simulink model "zd_model"  (Simulink 4.00)
settings: Solver=ode45  SolverMode=SingleTasking  StartTime=0.0  StopTime=T  FixedStep=.001  RelTol=1e-5  AbsTol=1e-6
values from neighbouring files (symbols this model uses):
  z0 = zd_project(x0)    [main_zd.m]    (also in sim_zd_cc.m = zd_project_cc(x0(1:10)'))
undefined symbols (not defined in the file or in its folder): x_0
settings Model: Creator=ewesterv  LastModifiedBy=ewesterv  TimeSaveName=t  LimitDataPoints=off  BlockReductionOpt=off

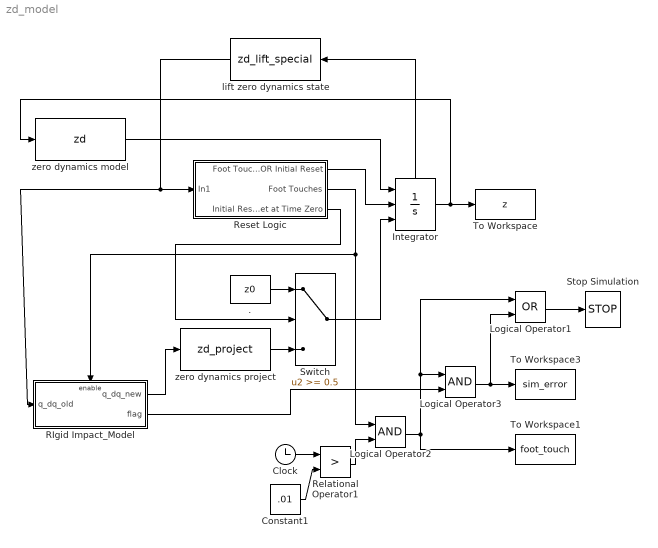
== system zd_model ==
  . : Constant  Value=z0
  Clock : Clock
      settings: DisplayTime=off  Decimation=10
  Constant1 : Constant  Value=.01
  Integrator : Integrator  ExternalReset=rising  InitialConditionSource=external  InitialCondition=x_0  LimitOutput=off  UpperSaturationLimit=inf  LowerSaturationLimit=-inf  ShowSaturationPort=off  ShowStatePort=on  AbsoluteTolerance=auto
  Logical Operator1 : Logic  Operator=OR  Inputs=2
  Logical Operator2 : Logic  Operator=AND  Inputs=2
  Logical Operator3 : Logic  Operator=AND  Inputs=2
  RIgid Impact_Model : Subsystem  TreatAsAtomicUnit=on
      settings: RTWFcnNameOpts=Auto  RTWFileNameOpts=Auto
  Relational Operator1 : RelationalOperator  Operator=>
  Reset Logic : Subsystem
      settings: RTWFcnNameOpts=Auto  RTWFileNameOpts=Auto
  Stop Simulation : Stop
  Switch : Switch  Threshold=0.5
  To Workspace : ToWorkspace  VariableName=z  SampleTime=-1  SaveFormat=Array
  To Workspace1 : ToWorkspace  VariableName=foot_touch  SampleTime=-1  SaveFormat=Array
  To Workspace3 : ToWorkspace  VariableName=sim_error  SampleTime=-1  SaveFormat=Array
  lift zero dynamics state : MATLABFcn  Orientation=left  MATLABFcn=zd_lift_special  OutputDimensions=10  OutputSignalType=auto  Output1D=off
  zero dynamics model : MATLABFcn  MATLABFcn=zd  OutputDimensions=2  OutputSignalType=auto  Output1D=on
  zero dynamics project : MATLABFcn  MATLABFcn=zd_project  OutputDimensions=2  OutputSignalType=auto  Output1D=on
  wires:
  Relational Operator1/1 -> Logical Operator2/2
  RIgid Impact_Model/2(flag) -> Logical Operator3/2
  Clock/1 -> Relational Operator1/1
  Integrator/1 -> To Workspace/1, zero dynamics model/1
  Reset Logic/2(Foot Touches) -> Logical Operator2/1, RIgid Impact_Model/Enable
  ./1 -> Switch/1
  Reset Logic/3(Initial Reset at Time Zero) -> Switch/2
  Switch/1 -> Integrator/3
  Reset Logic/1(Foot Touch OR Initial Reset) -> Integrator/2
  zero dynamics model/1 -> Integrator/1
  Constant1/1 -> Relational Operator1/2
  Logical Operator3/1 -> To Workspace3/1, Logical Operator1/2
  Integrator/State -> lift zero dynamics state/1
  lift zero dynamics state/1 -> Reset Logic/1(In1), RIgid Impact_Model/1(q_dq_old)
  RIgid Impact_Model/1(q_dq_new) -> zero dynamics project/1
  zero dynamics project/1 -> Switch/3
  Logical Operator1/1 -> Stop Simulation/1
  Logical Operator2/1 -> Logical Operator1/1, Logical Operator3/1, To Workspace1/1

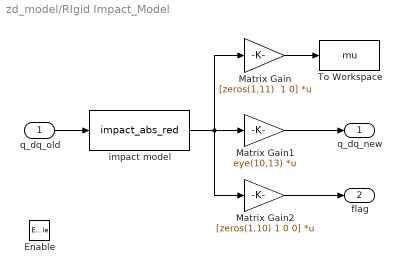
== system zd_model/RIgid Impact_Model ==
  q_dq_old : Inport  Port=1
  Enable : EnablePort
  Matrix Gain : Gain  Gain="[zeros(1,11)  1 0]"  Multiplication=Matrix(K*u)  SaturateOnIntegerOverflow=on
  Matrix Gain1 : Gain  Gain=eye(10,13)  Multiplication=Matrix(K*u)  SaturateOnIntegerOverflow=on
  Matrix Gain2 : Gain  Gain=[zeros(1,10) 1 0 0]  Multiplication=Matrix(K*u)  SaturateOnIntegerOverflow=on
  To Workspace : ToWorkspace  VariableName=mu  SampleTime=-1  SaveFormat=Array
  impact model : MATLABFcn  MATLABFcn=impact_abs_red  OutputDimensions=13  OutputSignalType=auto  Output1D=off
  q_dq_new : Outport  Port=1  InitialOutput=0
  flag : Outport  Port=2  InitialOutput=0
  wires:
  q_dq_old/1 -> impact model/1
  Matrix Gain1/1 -> q_dq_new/1
  Matrix Gain2/1 -> flag/1
  impact model/1 -> Matrix Gain1/1, Matrix Gain/1, Matrix Gain2/1
  Matrix Gain/1 -> To Workspace/1

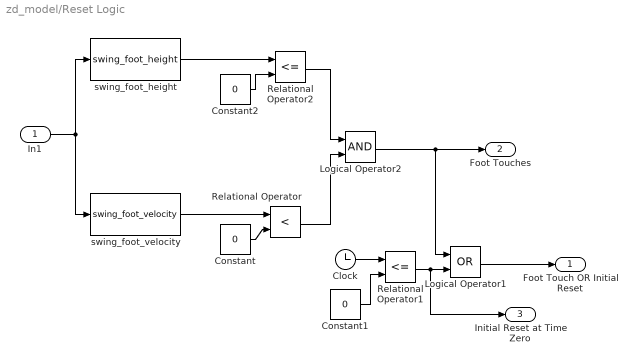
== system zd_model/Reset Logic ==
  In1 : Inport  Port=1
  Clock : Clock
      settings: DisplayTime=off  Decimation=10
  Constant : Constant  Value=0
  Constant1 : Constant  Value=0
  Constant2 : Constant  Value=0
  Logical Operator1 : Logic  Operator=OR  Inputs=2
  Logical Operator2 : Logic  Operator=AND  Inputs=2
  Relational Operator : RelationalOperator  Operator=<
  Relational Operator1 : RelationalOperator  Operator=<=
  Relational Operator2 : RelationalOperator  Operator=<=
  swing_foot_height : MATLABFcn  MATLABFcn=swing_foot_height  OutputDimensions=1  OutputSignalType=auto  Output1D=off
  swing_foot_velocity : MATLABFcn  MATLABFcn=swing_foot_velocity  OutputDimensions=1  OutputSignalType=auto  Output1D=off
  Foot Touch OR Initial Reset : Outport  Port=1  InitialOutput=0
  Foot Touches : Outport  Port=2  InitialOutput=0
  Initial Reset at Time Zero : Outport  Port=3  InitialOutput=0
  wires:
  Constant/1 -> Relational Operator/2
  Logical Operator1/1 -> Foot Touch OR Initial Reset/1
  Clock/1 -> Relational Operator1/1
  Constant1/1 -> Relational Operator1/2
  Relational Operator1/1 -> Logical Operator1/2, Initial Reset at Time Zero/1
  In1/1 -> swing_foot_height/1, swing_foot_velocity/1
  Constant2/1 -> Relational Operator2/2
  swing_foot_height/1 -> Relational Operator2/1
  swing_foot_velocity/1 -> Relational Operator/1
  Relational Operator2/1 -> Logical Operator2/1
  Relational Operator/1 -> Logical Operator2/2
  Logical Operator2/1 -> Logical Operator1/1, Foot Touches/1
